simulink model "LineCoding"  (R2023a)
settings: Solver=VariableStepAuto  StartTime=0.0  StopTime=16  RelTol=1e-3
libraries: commutil2 x2, commrandsrc3 x1, dspmathops x1
settings Model: Creator=gupta  LastModifiedBy=gupta

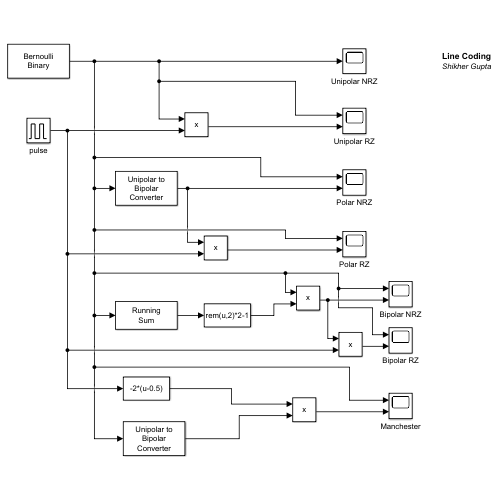
[thumbnail: Simulink's stored preview of the top-level diagram]
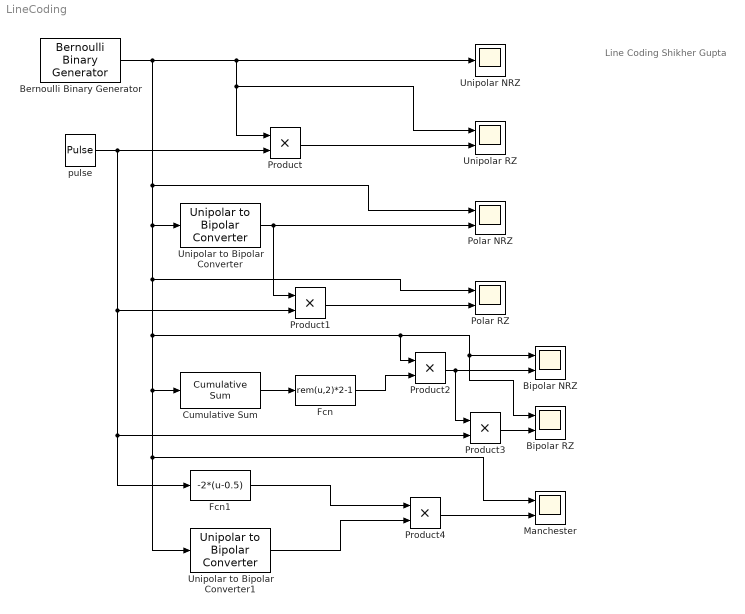
== system LineCoding ==
  note: Line Coding
      | Shikher Gupta
  Bernoulli Binary Generator : commrandsrc3/Bernoulli Binary Generator  ProbabilityOfZero=0.5  SeedSource=Auto  Seed=0  SampleTime=1  SamplesPerFrame=1  OutputDataType=double  SimulateUsing=Interpreted execution
  Bipolar NRZ : Scope  NumInputPorts=2
  Bipolar RZ : Scope  NumInputPorts=2
  Cumulative Sum : dspmathops/Cumulative Sum  dim=Channels (running sum)  InputProcessing=Columns as channels (frame based)  reset_popup=None  roundingMode=Floor  overflowMode=off  outputDataTypeStr=Inherit: Same as accumulator  outputMin=[]  outputMax=[]  outputLastDataTypeStr=Inherit: Same as accumulator
  Fcn : Fcn  Expr=rem(u,2)*2-1
  Fcn1 : Fcn  Expr=-2*(u-0.5)
  Manchester : Scope  NumInputPorts=2
  Polar NRZ : Scope  NumInputPorts=2
  Polar RZ : Scope  NumInputPorts=2
  Product{,1..4} (5 alike) : Product
  Unipolar NRZ : Scope
  Unipolar RZ : Scope  NumInputPorts=2
  Unipolar to Bipolar Converter : commutil2/Unipolar to Bipolar Converter  M=2  polarity=Positive  dataType=Inherit via internal rule
  Unipolar to Bipolar Converter1 : commutil2/Unipolar to Bipolar Converter  M=2  polarity=Positive  dataType=Inherit via internal rule
  pulse : DiscretePulseGenerator  PulseType=Time based  Period=1  PulseWidth=50
  wires:
  Bernoulli Binary Generator/1 -> Unipolar RZ/1, Product/1, Unipolar NRZ/1, Cumulative Sum/1, Manchester/1, Unipolar to Bipolar Converter1/1, Product2/1, Bipolar RZ/1, Bipolar NRZ/1, Polar RZ/1, Unipolar to Bipolar Converter/1, Polar NRZ/1
  pulse/1 -> Product/2, Fcn1/1, Product3/2, Product1/2
  Product/1 -> Unipolar RZ/2
  Unipolar to Bipolar Converter/1 -> Product1/1, Polar NRZ/2
  Product1/1 -> Polar RZ/2
  Cumulative Sum/1 -> Fcn/1
  Product2/1 -> Product3/1, Bipolar NRZ/2
  Fcn/1 -> Product2/2
  Product3/1 -> Bipolar RZ/2
  Fcn1/1 -> Product4/1
  Unipolar to Bipolar Converter1/1 -> Product4/2
  Product4/1 -> Manchester/2
